simulink model "Vehicle_model_sim"  (R2022b)
settings: Solver=FixedStepDiscrete  StartTime=0.0  StopTime=10  FixedStep=Ts  RelTol=1e-3  EnableMultiTasking=on
values from neighbouring files (symbols this model uses):
  L = 0.256    [Run_file.m]
  omegam0 = 0.0    (= 0)    [Run_file.m]
  rg = 9.49    [Run_file.m]
  Rw = 0.024    [Run_file.m]
  sat_pwm = 0.2    [Run_file.m]
  sat_steering = pi/6    (= 0.523598775598)    [Run_file.m]
  Ts = 0.01    [Run_file.m]
  V0 = [0.0; 0.0; 0.0]    [Run_file.m]
  X0 = [0.0; 0.0; 0.0]    [Run_file.m]
undefined symbols (not defined in the file or in its folder): Theta1, Theta2, Theta3, Theta4, Theta5
settings Model: Creator=RASLab-Distributed  LastModifiedBy=RASLab-Distributed
settings SolverCC: ConcurrentTasks=on  AlgebraicLoopSolver=TrustRegion  PositivePriorityOrder=on  InsertRTBMode=Never (minimum delay)
settings DataIOCC: SaveFormat=Array  SaveState=on  SignalLoggingName=logsOut
settings OptimizationCC: BlockReduction=off  BooleanDataType=off  OptimizeBlockIOStorage=off  BufferReuse=off  GlobalBufferReuse=off  ExpressionFolding=off  LocalBlockOutputs=off  InitFltsAndDblsToZero=on  OptimizeDataStoreBuffers=off  BusAssignmentInplaceUpdate=off
settings DebuggingCC: SaveWithParameterizedLinksMsg=none  UnderspecifiedInitializationDetection=Classic  MergeDetectMultiDrivingBlocksExec=none  CheckExecutionContextPreStartOutputMsg=on  SignalResolutionControl=TryResolveAllWithWarning  TasksWithSamePriorityMsg=none  UnconnectedInputMsg=warning  UnconnectedOutputMsg=warning  UnconnectedLineMsg=warning  SFUnexpectedBacktrackingDiag=warning  SFNoUnconditionalDefaultTransitionDiag=warning  SFExecutionAtInitializationDiag=none  SFMachineParentedDataDiag=warning  ArithmeticOperatorsInVariantConditions=warning
settings HardwareCC: ProdBitPerLong=64  ProdLongLongMode=on  ProdHWDeviceType=Intel->x86-64 (Linux 64)  TargetBitPerPointer=64  TargetBitPerSizeT=64  TargetBitPerPtrDiffT=64  TargetLongLongMode=on  TargetIntDivRoundTo=Zero  TargetEndianess=LittleEndian  TargetWordSize=64  TargetHWDeviceType=MATLAB Host
settings ModelReferenceCC: EnableRefExpFcnMdlSchedulingChecks=on  PropagateSignalLabelsOutOfModel=off
settings SFSimCC: SimUseLocalCustomCode=off  SimTargetLang=C++
settings RTWCC: Description=Simulink Real-Time  SystemTargetFile=slrealtime.tlc  TemplateMakefile=slrealtime_default_tmf  RTWUseLocalCustomCode=off  Toolchain=Simulink Real-Time Toolchain  BuildConfiguration=Faster Runs  CodeExecutionProfiling=on  TargetLang=C++  DLArmComputeVersion=19.05
settings CodeAppCC: StateflowObjectComments=on
settings ConfigComp: CovMetricSettings=dw  CovSaveCumulativeToWorkspaceVar=on  CovSaveSingleToWorkspaceVar=on  CovExternalEMLEnable=off  CovSFcnEnable=off

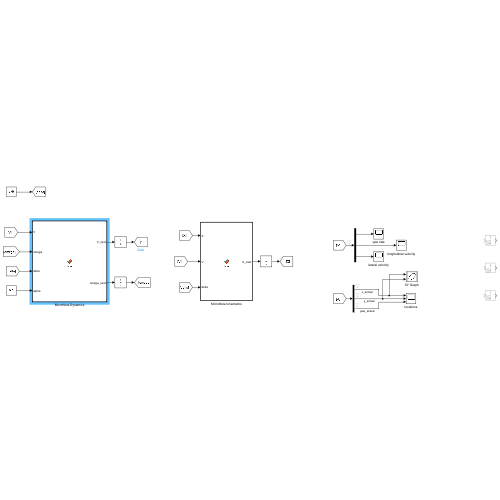
[thumbnail: Simulink's stored preview of the top-level diagram]
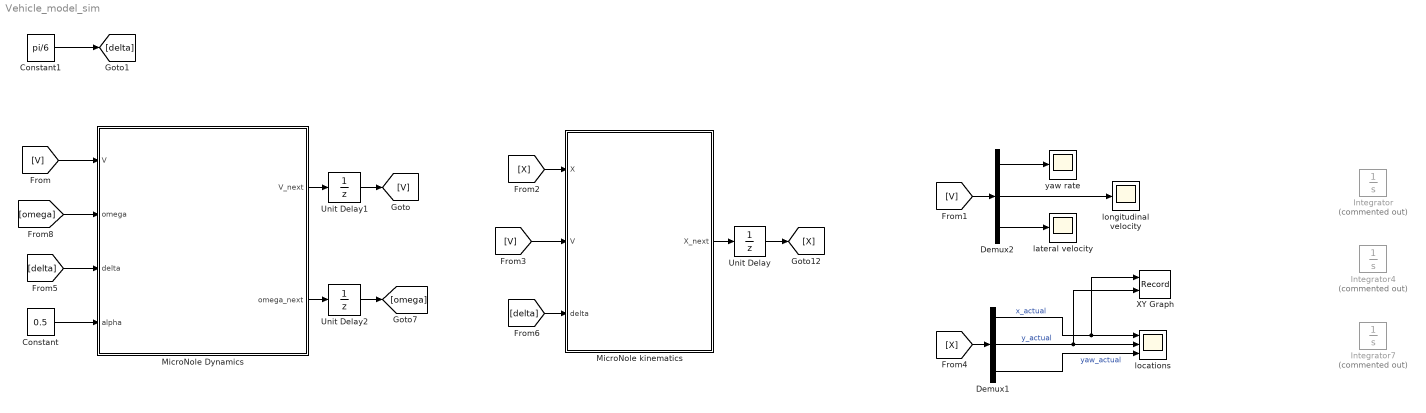
== system Vehicle_model_sim ==
  Constant : Constant  Value=0.5
  Constant1 : Constant  Value=pi/6
  Demux1 : Demux  Outputs=3
  Demux2 : Demux  Outputs=3
  Integrator : Integrator  Commented=on  InitialCondition=X0
  Integrator4 : Integrator  Commented=on  InitialCondition=V0
  Integrator7 : Integrator  Commented=on  InitialCondition=omegam0
  MicroNole Dynamics : MATLAB Function  TreatAsAtomicUnit=on
  MicroNole kinematics : MATLAB Function  TreatAsAtomicUnit=on
  Unit Delay : UnitDelay  InitialCondition=X0  SampleTime=Ts  HasFrameUpgradeWarning=on
  Unit Delay1 : UnitDelay  InitialCondition=V0  SampleTime=Ts  HasFrameUpgradeWarning=on
  Unit Delay2 : UnitDelay  InitialCondition=omegam0  SampleTime=Ts  HasFrameUpgradeWarning=on
  XY Graph : Record  FileSettingsInternal="{\"entries\":[{\"content\":{\"excelSettings\":{\"content\":{},\"type\":\"Streamout.ExcelSettings\"}},\"type\":\"Streamout.FileSettingStorage\",\"uuid\":\"6af3d020-c1a9-4012-bceb-3461c6254f57\"}],\"packageUris\":[\"http://schema.mathworks.com/mf0/streamout_blocks/R2020a\"],\"version\":\"1.0\"}"  Layout=[1 1]  SignalsInternal="{\"entries\":[{\"content\":{\"signals\":[{\"content\":{\"blockPath\":[\"Vehicle_model_sim/XY Graph\"],\"channel\":[],\"dimensions\":[1,1],\"domain\":\"Vehicle_model_sim/XY Graph\",\"lineColor\":\"#a2142f\",\"plots\":[1],\"port\":1,\"sid\":[\"\"],\"signalID\":2103,\"signalName\":\"x_actual\"},\"type\":\"RecordBlkView.Signal\",\"uuid\":\"ec722d5f-0a4c-43ac-8c46-c08fb54e5199\"},{\"content\":{\"blockPath\":[\"Vehicle_model_sim/XY Graph\"],\"channel\":[],\"dimensions\":[1,1],\"domain\":\"Vehicle_model_sim/XY Graph\",\"lineColor\":\"#139fff\",\"plots\":[1],\"port\":2,\"sid\":[\"\"],\"signalID\":2107,\"signalName\":\"y_actual\"},\"type\":\"RecordBlkView.Signal\",\"uuid\":\"39d7d27a-b0f4-4216-aa65-740f4a0b3f6d\"}]},\"type\":\"RecordBlkView.InputSignals\",\"uuid\":\"d3901b62-9cb2-4cd6-91e3-652dbe188164\"}],\"packageUris\":[\"http://schema.mathworks.com/mf0/streamout_blocks/R2020a\"],\"version\":\"1.0\"}"  VisualizationBindings="{\"xyplotplugin\":{\"info\":[{\"series\":[{\"bindingParametersList\":[{\"parameter\":\"X-Axis\",\"signalID\":2103,\"signalName\":\"x_actual\"},{\"parameter\":\"Y-Axis\",\"signalID\":2107,\"signalName\":\"y_actual\"}],\"seriesID\":54850}],\"subplotID\":1}]}}"  CompatibilityTag=XY
  lateral velocity : Scope
  locations : Scope  NumInputPorts=3
  longitudinal velocity : Scope
  yaw rate : Scope
  wires:
  [V] -> MicroNole Dynamics/1(V)
  Constant/1 -> MicroNole Dynamics/4(alpha)
  [X] -> MicroNole kinematics/1(X)
  [omega] -> MicroNole Dynamics/2(omega)
  Demux2/2 -> longitudinal velocity/1
  Demux2/1 -> yaw rate/1
  [V] -> Demux2/1
  Demux2/3 -> lateral velocity/1
  [X] -> Demux1/1
  Demux1/2 -> XY Graph/2, locations/2  "y_actual"
  Demux1/1 -> XY Graph/1, locations/1  "x_actual"
  Demux1/3 -> locations/3  "yaw_actual"
  MicroNole Dynamics/2(omega_next) -> Unit Delay2/1
  Unit Delay2/1 -> [omega]
  MicroNole Dynamics/1(V_next) -> Unit Delay1/1
  Unit Delay1/1 -> [V]
  MicroNole kinematics/1(X_next) -> Unit Delay/1
  Unit Delay/1 -> [X]
  [V] -> MicroNole kinematics/2(V)
  Constant1/1 -> [delta]
  [delta] -> MicroNole Dynamics/3(delta)
  [delta] -> MicroNole kinematics/3(delta)

== matlab function Vehicle_model_sim/MicroNole Dynamics ==
  data: V input; V_next output; omega input; delta input; alpha input; omega_next output; Theta2 parameter; Theta3 parameter; Theta4 parameter; L parameter; Rw parameter; rg parameter; Theta1 parameter; Theta5 parameter; sat_pwm parameter; sat_steering parameter; Ts parameter
% function [X_dot, V_dot, omega_dot] = fcn(X, V, omega, delta,alpha, Theta2, Theta3, Theta4, L, Rw, rg, Theta1, Theta5,sat_pwm, sat_steering)
function [V_next, omega_next] = fcn(V, omega, delta,alpha, Theta2, Theta3, Theta4, L, Rw, rg, Theta1, Theta5,sat_pwm, sat_steering,Ts)
%%
% States:
%        - X: [x,y,heading] world frame
%        - V: [Vx, Vy, yaw rate] car frame
%        - yaw: car yaw angle
%        - omega: motor rotation speed
% Inputs: 
%        - delta: steering angle
%        - alpha: throttle command (PWM%)
% parameters:
%

%% command satuation
if abs(alpha) > sat_pwm
    alpha =  sign(alpha) * sat_pwm;
end
if abs(delta) > sat_steering
    delta =  sign(delta) * sat_steering;
end
%% upacking inputs
yaw_rate = V(1);
Vx = V(2);
Vy = V(3);


%% dynamical model
Theta6 = Theta3*Theta5/Theta4;

omega_dot = -Theta1 * omega + Theta2 * alpha;
omega_next = omega + omega_dot*Ts;

A1 = (L/2) * Theta3 * delta * cos(delta);
B1 = (L/2) * Theta3 *(1-cos(delta));
C1 = ((1/2) * Theta3 * (1+cos(delta)) + Theta4) * (1/2) * L^2;
D1 = (Rw*L/(2*rg)) * Theta4 * sin(delta);
yaw_rate_dot = -C1*yaw_rate + A1*Vx + B1*Vy + D1*omega;

A2 = 2 * Theta5 + Theta6 * delta * sin(delta);
B2 = Theta6 * sin(delta);
C2 = L*Theta6*sin(delta)/2;
D2 = Theta5*Rw*(1+cos(delta))/rg;
Vx_dot = -A2*Vx + B2*Vy + C2*yaw_rate + yaw_rate*Vy + D2*omega;

A3 = Theta6 * delta * cos(delta);
B3 = Theta6 * (1+cos(delta));
C3 = L*(Theta6*(1-cos(delta))-2*Theta5)/2;
D3 = Theta5 * Rw *sin(delta)/rg;
Vy_dot = -B3*Vy + A3*Vx + C3*yaw_rate - yaw_rate*Vx + D3*omega;


%% packing outputs
V_dot = [yaw_rate_dot;
         Vx_dot;
         Vy_dot];
V_next = V + V_dot*Ts;

== matlab function Vehicle_model_sim/MicroNole kinematics ==
  data: X input; V input; X_next output; delta input; L parameter; Ts parameter
function X_next = fcn(X,V,delta,L,Ts)

%% unpack inputs
Vx = V(2);
Vy = V(3);

Phi = X(3);

%% forward kinematics (bickycle)
v = sqrt(Vx^2 + Vy^2);
beta = atan(tan(delta)/2);

x_dot = v * cos(Phi + beta);
y_dot = v * sin(Phi + beta);
Phi_dot = v * cos(beta) * tan(delta) / L;


X_dot = [x_dot;
         y_dot;
         Phi_dot];

X_next = X + X_dot*Ts;
